simulink model "sampleModel7126_pp_difftest"  (R2018a)
settings: Solver=VariableStepAuto  StartTime=0.0  StopTime=10.0  RelTol=1e-3
undefined symbols (not defined in the file or in its folder): DiscIntNeverNeededParam
libraries: simulink x367
(part 1 of 8)
settings Model: Creator=cyfuzz  LastModifiedBy=verivitallab
settings CodeAppCC: StateflowObjectComments=on

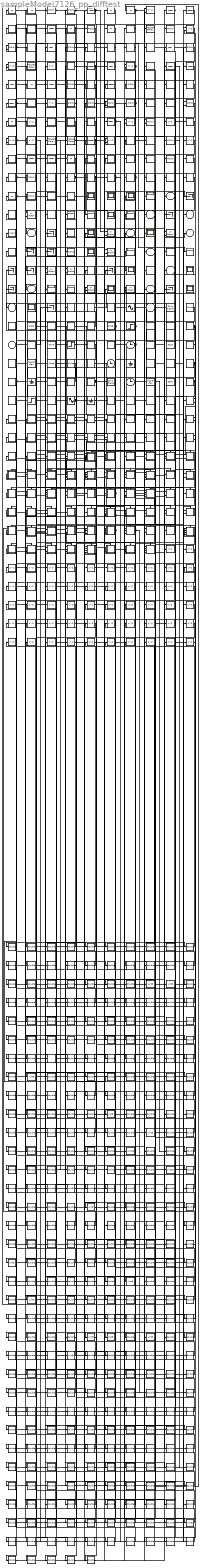
== system sampleModel7126_pp_difftest ==
  cfblk168 : Inport
  cfblk181 : Inport  Port=2
  cfblk{1..2,6..7,14,16,42,61,84,101} (10 alike) : UnitDelay
  cfblk{10,13,35,43,46,51,75,83} (8 alike) : DiscreteFilter  SampleTime=1
  cfblk{22,81,90,96..97,99..100,104} (8 alike) : simulink/Discrete/Difference  ICPrevInput=0.0  OutMin=[]  OutMax=[]  OutDataTypeStr=double  OutputDataTypeScalingMode=double  OutDataType=fixdt(1, 16)  OutScaling=2^-10  DoSatur=off
  cfblk{21,44,56,60,68,92,102} (7 alike) : simulink/Continuous/PID Controller (2DOF)  Controller=PID  TimeDomain=Discrete-time  SampleTime=1  IntegratorMethod=Forward Euler  FilterMethod=Forward Euler  Form=Parallel  UseFilter=on  ControllerParametersSource=internal  P=1  I=1  D=0  N=100  b=1  c=1  InitialConditionSource=internal  InitialConditionForIntegrator=0  InitialConditionForFilter=0  ExternalReset=none  LimitOutput=off  UpperSaturationLimit=inf  LowerSaturationLimit=-inf  LinearizeAsGain=off  AntiWindupMode=none  Kb=1  TrackingMode=off  Kt=1  PParamMin=[]  PParamMax=[]  IParamMin=[]  IParamMax=[]  DParamMin=[]  DParamMax=[]  NParamMin=[]  NParamMax=[]  bParamMin=[]  bParamMax=[]  cParamMin=[]  cParamMax=[]  KbParamMin=[]  KbParamMax=[]  KtParamMin=[]  KtParamMax=[]  POutMin=[]  POutMax=[]  IOutMin=[]  IOutMax=[]  DOutMin=[]  DOutMax=[]  NOutMin=[]  NOutMax=[]  bOutMin=[]  bOutMax=[]  cOutMin=[]  cOutMax=[]  KbOutMin=[]  KbOutMax=[]  KtOutMin=[]  KtOutMax=[]  IntegratorOutMin=[]  IntegratorOutMax=[]  FilterOutMin=[]  FilterOutMax=[]  SumOutMin=[]  SumOutMax=[]  Sum1OutMin=[]  Sum1OutMax=[]  Sum2OutMin=[]  Sum2OutMax=[]  Sum3OutMin=[]  Sum3OutMax=[]  SumI1OutMin=[]  SumI1OutMax=[]  SumI2OutMin=[]  SumI2OutMax=[]  SumI3OutMin=[]  SumI3OutMax=[]  SumDOutMin=[]  SumDOutMax=[]  SaturationOutMin=[]  SaturationOutMax=[]  IntegratorContinuousStateAttributes=''  IntegratorStateMustResolveToSignalObject=off  IntegratorRTWStateStorageClass=Auto  FilterContinuousStateAttributes=''  FilterStateMustResolveToSignalObject=off  FilterRTWStateStorageClass=Auto  DifferentiatorICPrevScaledInput=0  DifferentiatorOutMin=[]  DifferentiatorOutMax=[]  FilterDiffOutCoefMin=[]  FilterDiffOutCoefMax=[]  SumDenOutMin=[]  SumDenOutMax=[]  SumNumOutMin=[]  SumNumOutMax=[]  ReciprocalOutMin=[]  ReciprocalOutMax=[]  DivideOutMin=[]  DivideOutMax=[]  TunerSelectOption=Transfer Function Based (PID Tuner App)
  cfblk{25,52,58..59,64,103} (6 alike) : simulink/Discrete/Transfer Fcn Real Zero  ZeroZ=0.75  ICPrevInput=0.0  DoSatur=off
      settings: SourceProductName=Simulink  SourceProductBaseCode=SL
  cfblk{105..107,116,125,128,135,147,150,156,160,162} (12 alike) : Scope
      cfblk105 settings: Floating=on
      cfblk106 settings: Floating=on
      cfblk116 settings: Floating=on
      cfblk135 settings: Floating=on
      cfblk150 settings: Floating=on
      cfblk160 settings: Floating=on
      cfblk162 settings: Floating=on
  cfblk{108,114..115,117,137,140,153..154} (8 alike) : Display
  cfblk{11,27,45,49,85,93,95} (7 alike) : DiscreteStateSpace
  cfblk{110,119,123,132..133,141..142,146,151,159,163} (11 alike) : Terminator
  cfblk111 : ToWorkspace  VariableName=hcmzdjv  SaveFormat=Timeseries  SampleTime=-1
  cfblk{112,126,129,136,143..144,155,157} (8 alike) : simulink/Sinks/XY Graph  xmin=-1  xmax=1  ymin=-1  ymax=1  st=-1
  cfblk113 : ToWorkspace  VariableName=btwpcto  SaveFormat=Timeseries  SampleTime=-1
  cfblk{12,28,48,50,63,65,86,98} (8 alike) : DiscreteFir  SampleTime=1
  cfblk121 : ToWorkspace  VariableName=fvxrevr  SaveFormat=Timeseries  SampleTime=-1
  cfblk124 : ToWorkspace  VariableName=pxfsena  SaveFormat=Timeseries  SampleTime=-1
  cfblk131 : ToWorkspace  VariableName=uhzxskx  SaveFormat=Timeseries  SampleTime=-1
  cfblk134 : ToWorkspace  VariableName=rrjtpng  SaveFormat=Timeseries  SampleTime=-1
  cfblk139 : ToWorkspace  VariableName=kmkecre  SaveFormat=Timeseries  SampleTime=-1
  cfblk145 : ToWorkspace  VariableName=hvmekia  SaveFormat=Timeseries  SampleTime=-1
  cfblk148 : ToWorkspace  VariableName=eadgrso  SaveFormat=Timeseries  SampleTime=-1
  cfblk{3..4,15,19,24,30,47,54..55,57,79,89} (12 alike) : simulink/Continuous/PID Controller  Controller=PID  TimeDomain=Discrete-time  SampleTime=1  IntegratorMethod=Forward Euler  FilterMethod=Forward Euler  Form=Parallel  UseFilter=on  ControllerParametersSource=internal  P=1  I=1  D=0  N=100  InitialConditionSource=internal  InitialConditionForIntegrator=0  InitialConditionForFilter=0  ExternalReset=none  LimitOutput=off  UpperSaturationLimit=inf  LowerSaturationLimit=-inf  LinearizeAsGain=off  AntiWindupMode=none  Kb=1  TrackingMode=off  Kt=1  PParamMin=[]  PParamMax=[]  IParamMin=[]  IParamMax=[]  DParamMin=[]  DParamMax=[]  NParamMin=[]  NParamMax=[]  KbParamMin=[]  KbParamMax=[]  KtParamMin=[]  KtParamMax=[]  POutMin=[]  POutMax=[]  IOutMin=[]  IOutMax=[]  DOutMin=[]  DOutMax=[]  NOutMin=[]  NOutMax=[]  KbOutMin=[]  KbOutMax=[]  KtOutMin=[]  KtOutMax=[]  IntegratorOutMin=[]  IntegratorOutMax=[]  FilterOutMin=[]  FilterOutMax=[]  SumOutMin=[]  SumOutMax=[]  SumI1OutMin=[]  SumI1OutMax=[]  SumI2OutMin=[]  SumI2OutMax=[]  SumI3OutMin=[]  SumI3OutMax=[]  SumDOutMin=[]  SumDOutMax=[]  SaturationOutMin=[]  SaturationOutMax=[]  IntegratorContinuousStateAttributes=''  IntegratorStateMustResolveToSignalObject=off  IntegratorRTWStateStorageClass=Auto  FilterContinuousStateAttributes=''  FilterStateMustResolveToSignalObject=off  FilterRTWStateStorageClass=Auto  DifferentiatorICPrevScaledInput=0  DifferentiatorOutMin=[]  DifferentiatorOutMax=[]  FilterDiffOutCoefMin=[]  FilterDiffOutCoefMax=[]  SumDenOutMin=[]  SumDenOutMax=[]  SumNumOutMin=[]  SumNumOutMax=[]  ReciprocalOutMin=[]  ReciprocalOutMax=[]  DivideOutMin=[]  DivideOutMax=[]  TunerSelectOption=Transfer Function Based (PID Tuner App)
  cfblk164 : ToWorkspace  VariableName=thvkhab  SaveFormat=Timeseries  SampleTime=-1
  cfblk165 : simulink/Sources/Repeating Sequence Stair  OutValues=[3 1 4 2 1].'  tsamp=1  OutMin=[]  OutMax=[]  OutDataTypeStr=double  OutputDataTypeScalingMode=double  OutDataType=fixdt(0,8)  ConRadixGroup=Best Precision: Vector-wise  OutScaling=2^-12
  cfblk{166,174,180,213,216} (5 alike) : simulink/Sources/Repeating Sequence Interpolated  OutValues=[3 1 4 2 1].'  TimeValues=[0 0.1 0.5 0.6 1].'  LookUpMeth=Interpolation-Use End Values  tsamp=0.01  OutMin=[]  OutMax=[]  OutDataTypeStr=double  OutputDataTypeScalingMode=double  OutDataType=fixdt(0,8)  OutScaling=2^-10
  cfblk167 : Sin  SampleTime=0
  cfblk169 : simulink/Sources/Chirp Signal  f1=0.1  T=100  f2=1
  cfblk{17,38,87..88,91} (5 alike) : DiscreteZeroPole  Poles=[0 0.5]  Gain=1
  cfblk170 : DiscretePulseGenerator  PulseType=Time based  Period=10  PulseWidth=5
  cfblk{171,186,195,200,217} (5 alike) : simulink/Sources/Band-Limited White Noise  Cov=[0.1]  Ts=0.1  seed=[23341]
  cfblk172 : DigitalClock
  cfblk173 : RandomNumber  SampleTime=0.1
  cfblk{175,198..199,205,211} (5 alike) : simulink/Sources/Counter Free-Running  NumBits=16  tsamp=1
  cfblk176 : Constant  Value=0318  OutDataTypeStr=double  SampleTime=1
  cfblk177 : Step  After=82  SampleTime=0
  cfblk178 : simulink/Sources/Counter Limited  uplimit=7  tsamp=1
  cfblk179 : UniformRandomNumber  SampleTime=0.1
  cfblk{18,32,73..74} (4 alike) : simulink/Discrete/Tapped Delay  vinit=0.0  samptime=-1  NumDelays=1  DelayOrder=Oldest  includeCurrent=off
  cfblk182 : simulink/Sources/Repeating Sequence Stair  OutValues=[3 1 4 2 1].'  tsamp=1  OutMin=[]  OutMax=[]  OutDataTypeStr=double  OutputDataTypeScalingMode=double  OutDataType=fixdt(0,8)  ConRadixGroup=Best Precision: Vector-wise  OutScaling=2^-12
  cfblk183 : Constant  Value=5175  OutDataTypeStr=double  SampleTime=1
  cfblk184 : Step  After=84  SampleTime=0
  cfblk185 : simulink/Sources/Repeating Sequence  rep_seq_t=[0 2]  rep_seq_y=[0 2]
  cfblk187 : Clock
  cfblk188 : RandomNumber  SampleTime=0.1
  cfblk189 : Constant  Value=8152  OutDataTypeStr=double  SampleTime=1
  cfblk190 : simulink/Sources/Counter Limited  uplimit=7  tsamp=1
  cfblk191 : RandomNumber  SampleTime=0.1
  cfblk192 : SignalGenerator  Units=rad/sec
  cfblk193 : DiscretePulseGenerator  PulseType=Time based  Period=10  PulseWidth=5
  cfblk194 : DiscretePulseGenerator  PulseType=Time based  Period=10  PulseWidth=5
  cfblk196 : Clock
  cfblk197 : Ground
  cfblk20 : Delay  DelayLengthSource=Input port  SampleTime=1
      settings: InputPortMap=u0,p1
  cfblk201 : simulink/Sources/Repeating Sequence  rep_seq_t=[0 2]  rep_seq_y=[0 2]
  cfblk202 : Ground
  cfblk203 : simulink/Sources/Counter Limited  uplimit=7  tsamp=1
  cfblk204 : UniformRandomNumber  SampleTime=0.1
  cfblk206 : simulink/Sources/Chirp Signal  f1=0.1  T=100  f2=1
  cfblk207 : Clock
  cfblk208 : SignalGenerator  Units=rad/sec
  cfblk209 : Constant  Value=6334  OutDataTypeStr=double  SampleTime=1
  cfblk210 : UniformRandomNumber  SampleTime=0.1
  cfblk212 : Step  After=96  SampleTime=0
  cfblk214 : Sin  SampleTime=0
  cfblk215 : Ground
  cfblk{218..244} (27 alike) : If  SampleTime=1
  cfblk{23,29,36,41} (4 alike) : DiscreteIntegrator  OutDataTypeStr=double  ICPrevOutput=DiscIntNeverNeededParam  ICPrevScaledInput=DiscIntNeverNeededParam
  cfblk245 : Subsystem  TreatAsAtomicUnit=on
  cfblk246 : Subsystem  TreatAsAtomicUnit=on
  cfblk247 : Subsystem  TreatAsAtomicUnit=on
  cfblk248 : Subsystem  TreatAsAtomicUnit=on
  cfblk249 : Subsystem  TreatAsAtomicUnit=on
  cfblk250 : Subsystem  TreatAsAtomicUnit=on
  cfblk251 : Subsystem  TreatAsAtomicUnit=on
  cfblk252 : Subsystem  TreatAsAtomicUnit=on
  cfblk253 : Subsystem  TreatAsAtomicUnit=on
  cfblk254 : Subsystem  TreatAsAtomicUnit=on
  cfblk255 : Subsystem  TreatAsAtomicUnit=on
  cfblk256 : Subsystem  TreatAsAtomicUnit=on
  cfblk257 : Subsystem  TreatAsAtomicUnit=on
  cfblk258 : Subsystem  TreatAsAtomicUnit=on
  cfblk259 : Subsystem  TreatAsAtomicUnit=on
  cfblk{26,34,70,77} (4 alike) : simulink/Discrete/Transfer Fcn First Order  PoleZ=0.95  ICPrevOutput=0.0  DoSatur=off
      settings: SourceProductName=Simulink
  cfblk260 : Subsystem  TreatAsAtomicUnit=on
  cfblk261 : Subsystem  TreatAsAtomicUnit=on
  cfblk262 : Subsystem  TreatAsAtomicUnit=on
  cfblk263 : Subsystem  TreatAsAtomicUnit=on
  cfblk264 : Subsystem  TreatAsAtomicUnit=on
  cfblk265 : Subsystem  TreatAsAtomicUnit=on
  cfblk266 : Subsystem  TreatAsAtomicUnit=on
  cfblk267 : Subsystem  TreatAsAtomicUnit=on
  cfblk268 : Subsystem  TreatAsAtomicUnit=on
  cfblk269 : Subsystem  TreatAsAtomicUnit=on
  cfblk270 : Subsystem  TreatAsAtomicUnit=on
  cfblk271 : Subsystem  TreatAsAtomicUnit=on
  cfblk272 : Subsystem  TreatAsAtomicUnit=on
  cfblk273 : Subsystem  TreatAsAtomicUnit=on
  cfblk274 : Subsystem  TreatAsAtomicUnit=on
  cfblk275 : Subsystem  TreatAsAtomicUnit=on
  cfblk276 : Subsystem  TreatAsAtomicUnit=on
  cfblk277 : Subsystem  TreatAsAtomicUnit=on
  cfblk278 : Subsystem  TreatAsAtomicUnit=on
  cfblk279 : Subsystem  TreatAsAtomicUnit=on
  cfblk280 : Subsystem  TreatAsAtomicUnit=on
  cfblk281 : Subsystem  TreatAsAtomicUnit=on
  cfblk282 : Subsystem  TreatAsAtomicUnit=on
  cfblk283 : Subsystem  TreatAsAtomicUnit=on
  cfblk284 : Subsystem  TreatAsAtomicUnit=on
  cfblk285 : Subsystem  TreatAsAtomicUnit=on
  cfblk286 : Subsystem  TreatAsAtomicUnit=on
  cfblk287 : Subsystem  TreatAsAtomicUnit=on
  cfblk288 : Subsystem  TreatAsAtomicUnit=on
  cfblk289 : Subsystem  TreatAsAtomicUnit=on
  cfblk290 : Subsystem  TreatAsAtomicUnit=on
  cfblk291 : Subsystem  TreatAsAtomicUnit=on
  cfblk292 : Subsystem  TreatAsAtomicUnit=on
  cfblk293 : Subsystem  TreatAsAtomicUnit=on
  cfblk294 : Subsystem  TreatAsAtomicUnit=on
  cfblk295 : Subsystem  TreatAsAtomicUnit=on
  cfblk296 : Subsystem  TreatAsAtomicUnit=on
  cfblk297 : Subsystem  TreatAsAtomicUnit=on
  cfblk298 : Subsystem  TreatAsAtomicUnit=on
  cfblk{33,53,62,69,80,299..350} (57 alike) : Delay  SampleTime=1
  cfblk{31,37,67,72,76} (5 alike) : Delay  ShowEnablePort=on  SampleTime=1
      settings: InputPortMap=u0,e6
  cfblk{5,9,39..40,66,82} (6 alike) : DiscreteTransferFcn  SampleTime=1
  cfblk71 : Delay  DelayLengthSource=Input port  SampleTime=1
      settings: InputPortMap=u0,p1
  cfblk78 : simulink/Discrete/Transfer Fcn Lead or Lag  PoleZ=0.95  ZeroZ=0.75  ICPrevOutput=0.0  ICPrevInput=0.0  DoSatur=off
      settings: SourceProductName=Simulink  SourceProductBaseCode=SL
  cfblk8 : Delay  DelayLengthSource=Input port  SampleTime=1
      settings: InputPortMap=u0,p1
  cfblk94 : simulink/Discrete/Transfer Fcn Lead or Lag  PoleZ=0.95  ZeroZ=0.75  ICPrevOutput=0.0  ICPrevInput=0.0  DoSatur=off
      settings: SourceProductName=Simulink  SourceProductBaseCode=SL
  cyemi_{0..26,29..61,63..67,99..100,133,181,203..205,222..224,233,243,297..298,328..331,345..348,357..358,383..384,395..398,407,446..448,457,485..486,496..498,533..534,548,589,615,629..632,639..640,673..674,688..689,706,719..720,753,763,802..803,813..814,856..857,929..930,939,941,971..973,985..987,999..1000,1013..1014,1055..1057,1064..1065,1070..1072,1081..1082,1094,1133,1136..1137,1146,1154..1155,1186..1187,1202..1204,1216..1219,1266,1285..1287,1295,1297..1298,1340..1359,1362,1364..1367,1370..1409,1411..1430,1432..1464,1466..1480} (311 alike) : DataTypeConversion  OutDataTypeStr=double
  cyemi_{27..28,180,385,495,801,940,1063,1135,1267,1296,1360..1361,1363,1369,1410,1465} (17 alike) : DataTypeConversion  OutDataTypeStr=uint8
  cyemi_{616,707,804,1134,1431} (5 alike) : DataTypeConversion  OutDataTypeStr=uint16
  cyemi_1368 : DataTypeConversion  OutDataTypeStr=fixdt('ufix32_En8')
  cyemi_62 : DataTypeConversion  OutDataTypeStr=fixdt('ufix32_En8')
  cfblk109 : Outport
  cfblk118 : Outport  Port=2
  cfblk120 : Outport  Port=3
  cfblk122 : Outport  Port=4
  cfblk127 : Outport  Port=5
  cfblk130 : Outport  Port=6
  cfblk138 : Outport  Port=7
  cfblk149 : Outport  Port=8
  cfblk152 : Outport  Port=9
  cfblk158 : Outport  Port=10
  cfblk161 : Outport  Port=11
  wires:
  cfblk249/1(cfblk2) -> cfblk149/1
  cfblk21/1 -> cfblk147/1, cyemi_53/1
  cfblk182/1 -> cfblk163/1
  cfblk11/1 -> cfblk140/1
  cfblk269/2(cfblk7) -> cyemi_689/1, cyemi_1370/1, cyemi_1459/1
  cfblk34/1 -> cfblk118/1
  cfblk175/1 -> cfblk153/1
  cfblk13/1 -> cfblk119/1
  cfblk211/1 -> cfblk108/1
  cfblk4/1 -> cyemi_719/1, cyemi_814/1, cyemi_1441/1
  cfblk252/1(cfblk2) -> cyemi_1383/1, cyemi_1468/1
  cfblk286/1(cfblk2) -> cyemi_1360/1, cyemi_1369/1
  cfblk180/1 -> cyemi_1365/1, cyemi_1476/1
  cfblk23/1 -> cyemi_1136/1, cyemi_1397/1, cyemi_1406/1
  cfblk268/1(cfblk2) -> cfblk109/1
  cfblk282/1(cfblk2) -> cfblk123/1
  cfblk14/1 -> cyemi_99/1, cyemi_986/1
  cfblk75/1 -> cfblk110/1, cyemi_1409/1
  cfblk9/1 -> cyemi_534/1, cyemi_1392/1
  cfblk101/1 -> cfblk136/2, cyemi_1351/1
  cfblk51/1 -> cyemi_397/1, cyemi_1384/1, cyemi_1471/1
  cfblk95/1 -> cyemi_1376/1, cyemi_1442/1
  cfblk178/1 -> cyemi_385/1, cyemi_940/1
  cfblk37/1 -> cfblk112/1, cfblk126/2, cyemi_1347/1
  cfblk177/1 -> cyemi_1432/1, cyemi_1452/1
  cfblk254/1(cfblk2) -> cfblk144/1
  cfblk200/1 -> cyemi_17/1, cyemi_803/1
  cfblk268/3(cfblk13) -> cfblk130/1, cyemi_1402/1
  cfblk59/1 -> cyemi_25/1, cyemi_133/1
  cfblk87/1 -> cfblk115/1
  cfblk53/1 -> cyemi_14/1, cyemi_1344/1
  cfblk71/1 -> cyemi_37/1, cyemi_448/1, cyemi_1340/1
  cfblk188/1 -> cfblk159/1
  cfblk62/1 -> cfblk142/1
  cfblk73/1 -> cfblk129/2, cyemi_673/1
  cfblk66/1 -> cyemi_6/1, cyemi_31/1, cyemi_1440/1
  cfblk166/1 -> cfblk138/1
  cfblk3/1 -> cyemi_65/1, cyemi_1443/1
  cfblk7/1 -> cyemi_18/1, cyemi_56/1
  cfblk287/1(cfblk2) -> cyemi_3/1, cyemi_987/1, cyemi_1393/1
  cfblk266/1(cfblk2) -> cyemi_1378/1, cyemi_1379/1
  cfblk48/1 -> cyemi_589/1, cyemi_1380/1
  cfblk72/1 -> cyemi_1346/1, cyemi_1348/1
  cfblk278/1(cfblk2) -> cfblk107/1
  cfblk214/1 -> cfblk114/1, cyemi_331/1
  cfblk176/1 -> cyemi_1000/1, cyemi_1401/1
  cfblk263/2(cfblk14) -> cfblk143/1
  cfblk172/1 -> cyemi_486/1, cyemi_1297/1
  cfblk91/1 -> cfblk161/1, cyemi_222/1
  cfblk283/1(cfblk2) -> cfblk143/2
  cfblk100/1 -> cfblk112/2
  cfblk261/1(cfblk2) -> cfblk137/1
  cfblk277/2(cfblk17) -> cfblk125/1
  cfblk210/1 -> cyemi_1070/1, cyemi_1436/1
  cfblk187/1 -> cfblk141/1, cyemi_1341/1
  cfblk281/1(cfblk2) -> cfblk127/1
  cfblk205/1 -> cyemi_616/1, cyemi_804/1
  cfblk206/1 -> cfblk154/1
  cfblk57/1 -> cfblk122/1, cyemi_45/1
  cfblk5/1 -> cfblk126/1, cyemi_857/1
  cfblk64/1 -> cfblk132/1
  cfblk204/1 -> cfblk133/1
  cfblk253/1(cfblk2) -> cfblk158/1
  cfblk94/1 -> cyemi_15/1, cyemi_383/1
  cfblk39/1 -> cyemi_328/1, cyemi_497/1
  cfblk247/3(cfblk17) -> cfblk117/1
  cfblk35/1 -> cyemi_59/1, cyemi_498/1
  cfblk183/1 -> cyemi_396/1, cyemi_1056/1
  cfblk201/1 -> cyemi_447/1, cyemi_1014/1
  cfblk250/2(cfblk9) -> cyemi_1071/1, cyemi_1155/1
  cfblk280/3(cfblk12) -> cfblk155/1
  cfblk208/1 -> cyemi_630/1, cyemi_1420/1
  cfblk168/1 -> cyemi_348/1, cyemi_398/1
  cfblk248/2(cfblk17) -> cyemi_446/1, cyemi_1154/1
  cfblk83/1 -> cyemi_813/1, cyemi_1371/1
  cfblk25/1 -> cfblk136/1
  cfblk251/1(cfblk2) -> cfblk155/2
  cfblk79/1 -> cyemi_496/1, cyemi_1435/1
  cfblk276/3(cfblk13) -> cyemi_1134/1, cyemi_1431/1
  cfblk96/1 -> cyemi_330/1, cyemi_1472/1
  cfblk207/1 -> cfblk129/1
  cfblk15/1 -> cfblk152/1
  cfblk199/1 -> cfblk120/1
  cfblk165/1 -> cfblk157/1
  cfblk296/3(cfblk17) -> cfblk146/1
  cfblk97/1 -> cyemi_457/1, cyemi_1446/1
  cfblk289/2(cfblk8) -> cfblk157/2, cyemi_1394/1
  cfblk292/3(cfblk13) -> cfblk151/1, cyemi_243/1
  cfblk290/4(cfblk15) -> cfblk156/1
  cfblk283/4(cfblk17) -> cyemi_181/1, cyemi_1385/1
  cfblk264/3(cfblk14) -> cfblk128/1
  cfblk288/1(cfblk2) -> cyemi_1366/1, cyemi_1367/1
  cfblk297/2(cfblk10) -> cfblk144/2
  cfblk218/1 -> cfblk245/Action
  cfblk218/2 -> cfblk246/Action
  cfblk219/1 -> cfblk247/Action
  cfblk219/2 -> cfblk248/Action
  cfblk220/1 -> cfblk249/Action
  cfblk220/2 -> cfblk250/Action
  cfblk221/1 -> cfblk251/Action
  cfblk221/2 -> cfblk252/Action
  cfblk222/1 -> cfblk253/Action
  cfblk222/2 -> cfblk254/Action
  cfblk223/1 -> cfblk255/Action
  cfblk223/2 -> cfblk256/Action
  cfblk224/1 -> cfblk257/Action
  cfblk224/2 -> cfblk258/Action
  cfblk225/1 -> cfblk259/Action
  cfblk225/2 -> cfblk260/Action
  cfblk226/1 -> cfblk261/Action
  cfblk226/2 -> cfblk262/Action
  cfblk227/1 -> cfblk263/Action
  cfblk227/2 -> cfblk264/Action
  cfblk228/1 -> cfblk265/Action
  cfblk228/2 -> cfblk266/Action
  cfblk229/1 -> cfblk267/Action
  cfblk229/2 -> cfblk268/Action
  cfblk230/1 -> cfblk269/Action
  cfblk230/2 -> cfblk270/Action
  cfblk231/1 -> cfblk271/Action
  cfblk231/2 -> cfblk272/Action
  cfblk232/1 -> cfblk273/Action
  cfblk232/2 -> cfblk274/Action
  cfblk233/1 -> cfblk275/Action
  cfblk233/2 -> cfblk276/Action
  cfblk234/1 -> cfblk277/Action
  cfblk234/2 -> cfblk278/Action
  cfblk235/1 -> cfblk279/Action
  cfblk235/2 -> cfblk280/Action
  cfblk236/1 -> cfblk281/Action
  cfblk236/2 -> cfblk282/Action
  cfblk237/1 -> cfblk283/Action
  cfblk237/2 -> cfblk284/Action
  cfblk238/1 -> cfblk285/Action
  cfblk238/2 -> cfblk286/Action
  cfblk239/1 -> cfblk287/Action
  cfblk239/2 -> cfblk288/Action
  cfblk240/1 -> cfblk289/Action
  cfblk240/2 -> cfblk290/Action
  cfblk241/1 -> cfblk291/Action
  cfblk241/2 -> cfblk292/Action
  cfblk242/1 -> cfblk293/Action
  cfblk242/2 -> cfblk294/Action
  cfblk243/1 -> cfblk295/Action
  cfblk243/2 -> cfblk296/Action
  cfblk244/1 -> cfblk297/Action
  cfblk244/2 -> cfblk298/Action
  cyemi_0/1 -> cfblk1/1
  cfblk290/5(cfblk16) -> cyemi_0/1
  cyemi_1/1 -> cfblk10/1
  cfblk196/1 -> cyemi_1/1
  cyemi_2/1 -> cfblk100/1
  cfblk33/1 -> cyemi_2/1
  cyemi_3/1 -> cfblk101/1
  cyemi_4/1 -> cfblk102/1
  cfblk282/5(cfblk15) -> cyemi_4/1
  cyemi_5/1 -> cfblk102/2
  cfblk16/1 -> cyemi_5/1
  cyemi_6/1 -> cfblk103/1
  cyemi_7/1 -> cfblk104/1
  cfblk267/2(cfblk14) -> cyemi_7/1
  cyemi_8/1 -> cfblk11/1
  cfblk259/2(cfblk8) -> cyemi_8/1
  cyemi_9/1 -> cfblk111/1
  cfblk257/1(cfblk2) -> cyemi_9/1
  cyemi_10/1 -> cfblk113/1
  cfblk171/1 -> cyemi_10/1
  cyemi_11/1 -> cfblk12/1
  cfblk40/1 -> cyemi_11/1
  cyemi_12/1 -> cfblk121/1
  cfblk194/1 -> cyemi_12/1
  cyemi_13/1 -> cfblk124/1
  cfblk80/1 -> cyemi_13/1
  cyemi_14/1 -> cfblk13/1
  cyemi_15/1 -> cfblk131/1
  cyemi_16/1 -> cfblk134/1
  cfblk268/2(cfblk12) -> cyemi_16/1
  cyemi_17/1 -> cfblk139/1
  cyemi_18/1 -> cfblk14/1
  cyemi_19/1 -> cfblk145/1
  cfblk248/1(cfblk2) -> cyemi_19/1
  cyemi_20/1 -> cfblk148/1
  cfblk26/1 -> cyemi_20/1
  cyemi_21/1 -> cfblk15/1
  cfblk298/1(cfblk2) -> cyemi_21/1
  cyemi_22/1 -> cfblk16/1
  cfblk47/1 -> cyemi_22/1
  cyemi_23/1 -> cfblk164/1
  cfblk247/1(cfblk2) -> cyemi_23/1
  cyemi_24/1 -> cfblk17/1
  cfblk272/1(cfblk2) -> cyemi_24/1
  cyemi_25/1 -> cfblk18/1
  cyemi_26/1 -> cfblk19/1
  cfblk202/1 -> cyemi_26/1
  cyemi_27/1 -> cfblk2/1
  cfblk318/1 -> cyemi_27/1
  cyemi_28/1 -> cfblk20/1
  cfblk2/1 -> cyemi_28/1
  cyemi_29/1 -> cfblk20/2
  cfblk350/1 -> cyemi_29/1
  cyemi_30/1 -> cfblk21/1
  cfblk259/1(cfblk2) -> cyemi_30/1
  cyemi_31/1 -> cfblk21/2
  cyemi_32/1 -> cfblk218/1
  cfblk300/1 -> cyemi_32/1
  cyemi_33/1 -> cfblk219/1
  cfblk63/1 -> cyemi_33/1
  cyemi_34/1 -> cfblk22/1
  cfblk181/1 -> cyemi_34/1
  cyemi_35/1 -> cfblk220/1
  cfblk293/1(cfblk2) -> cyemi_35/1
  cyemi_36/1 -> cfblk221/1
  cfblk61/1 -> cyemi_36/1
  cyemi_37/1 -> cfblk222/1
  cyemi_38/1 -> cfblk223/1
  cfblk306/1 -> cyemi_38/1
  cyemi_39/1 -> cfblk224/1
  cfblk28/1 -> cyemi_39/1
  cyemi_40/1 -> cfblk225/1
  cfblk317/1 -> cyemi_40/1
  cyemi_41/1 -> cfblk226/1
  cfblk88/1 -> cyemi_41/1
  cyemi_42/1 -> cfblk227/1
  cfblk70/1 -> cyemi_42/1
  cyemi_43/1 -> cfblk228/1
  cfblk27/1 -> cyemi_43/1
  cyemi_44/1 -> cfblk229/1
  cfblk303/1 -> cyemi_44/1
  cyemi_45/1 -> cfblk23/1
  cyemi_46/1 -> cfblk230/1
  cfblk325/1 -> cyemi_46/1
  cyemi_47/1 -> cfblk231/1
  cfblk284/2(cfblk9) -> cyemi_47/1
  cyemi_48/1 -> cfblk232/1
  cfblk311/1 -> cyemi_48/1
  cyemi_49/1 -> cfblk233/1
  cfblk191/1 -> cyemi_49/1
  cyemi_50/1 -> cfblk234/1
  cfblk84/1 -> cyemi_50/1
  cyemi_51/1 -> cfblk235/1
  cfblk93/1 -> cyemi_51/1
  cyemi_52/1 -> cfblk236/1
  cfblk60/1 -> cyemi_52/1
  cyemi_53/1 -> cfblk237/1
  cyemi_54/1 -> cfblk238/1
  cfblk314/1 -> cyemi_54/1
  cyemi_55/1 -> cfblk239/1
  cfblk340/1 -> cyemi_55/1
  cyemi_56/1 -> cfblk24/1
  cyemi_57/1 -> cfblk240/1
  cfblk313/1 -> cyemi_57/1
  cyemi_58/1 -> cfblk241/1
  cfblk329/1 -> cyemi_58/1
  cyemi_59/1 -> cfblk242/1
  cyemi_60/1 -> cfblk243/1
  cfblk245/3(cfblk17) -> cyemi_60/1
  cyemi_61/1 -> cfblk244/1
  cfblk285/1(cfblk2) -> cyemi_61/1
  cyemi_62/1 -> cfblk245/1(cfblk1)
  cfblk322/1 -> cyemi_62/1
  cyemi_63/1 -> cfblk245/2(cfblk11)
  cfblk320/1 -> cyemi_63/1
  cyemi_64/1 -> cfblk245/3(cfblk12)
  cfblk260/2(cfblk10) -> cyemi_64/1
  cyemi_65/1 -> cfblk245/4(cfblk13)
  cyemi_66/1 -> cfblk245/5(cfblk14)
  cfblk333/1 -> cyemi_66/1
  cyemi_67/1 -> cfblk245/6(cfblk15)
  cfblk345/1 -> cyemi_67/1
  cyemi_99/1 -> cfblk246/1(cfblk1)
  cyemi_100/1 -> cfblk246/2(cfblk8)
  cfblk52/1 -> cyemi_100/1
  cyemi_133/1 -> cfblk247/1(cfblk1)
  cyemi_180/1 -> cfblk248/1(cfblk1)
  cfblk276/2(cfblk12) -> cyemi_180/1
  cyemi_181/1 -> cfblk248/2(cfblk16)
  cyemi_203/1 -> cfblk249/1(cfblk1)
  cfblk54/1 -> cyemi_203/1
  cyemi_204/1 -> cfblk249/2(cfblk14)
  cfblk10/1 -> cyemi_204/1
  cyemi_205/1 -> cfblk249/3(cfblk15)
  cfblk341/1 -> cyemi_205/1
  cyemi_222/1 -> cfblk25/1
  cyemi_223/1 -> cfblk250/1(cfblk1)
  cfblk184/1 -> cyemi_223/1
  cyemi_224/1 -> cfblk250/2(cfblk8)
  cfblk305/1 -> cyemi_224/1
  cyemi_233/1 -> cfblk251/1(cfblk1)
  cfblk292/2(cfblk12) -> cyemi_233/1
  cyemi_243/1 -> cfblk252/1(cfblk1)
  cyemi_297/1 -> cfblk253/1(cfblk1)
  cfblk261/2(cfblk12) -> cyemi_297/1
  cyemi_298/1 -> cfblk253/2(cfblk8)
  cfblk274/2(cfblk8) -> cyemi_298/1
  cyemi_328/1 -> cfblk254/1(cfblk1)
  cyemi_329/1 -> cfblk254/2(cfblk14)
  cfblk255/1(cfblk2) -> cyemi_329/1
  cyemi_330/1 -> cfblk254/3(cfblk15)
  cyemi_331/1 -> cfblk254/4(cfblk16)
  cyemi_345/1 -> cfblk255/1(cfblk1)
  cfblk343/1 -> cyemi_345/1
  cyemi_346/1 -> cfblk255/2(cfblk9)
  cfblk339/1 -> cyemi_346/1
  cyemi_347/1 -> cfblk255/3(cfblk10)
  cfblk267/1(cfblk2) -> cyemi_347/1
  cyemi_348/1 -> cfblk255/4(cfblk11)
  cyemi_357/1 -> cfblk256/1(cfblk1)
  cfblk330/1 -> cyemi_357/1
  cyemi_358/1 -> cfblk256/2(cfblk10)
  cfblk307/1 -> cyemi_358/1
  cyemi_383/1 -> cfblk257/1(cfblk1)
  cyemi_384/1 -> cfblk257/2(cfblk12)
  cfblk264/2(cfblk13) -> cyemi_384/1
  cyemi_385/1 -> cfblk257/3(cfblk13)
  cyemi_395/1 -> cfblk258/1(cfblk1)
  cfblk56/1 -> cyemi_395/1
  cyemi_396/1 -> cfblk258/2(cfblk8)
  cyemi_397/1 -> cfblk258/3(cfblk9)
  cyemi_398/1 -> cfblk258/4(cfblk10)
  cyemi_407/1 -> cfblk259/1(cfblk1)
  cfblk308/1 -> cyemi_407/1
  cyemi_446/1 -> cfblk26/1
  cyemi_447/1 -> cfblk260/1(cfblk1)
  cyemi_448/1 -> cfblk260/2(cfblk9)
  cyemi_457/1 -> cfblk261/1(cfblk1)
  cyemi_485/1 -> cfblk262/1(cfblk1)
  cfblk197/1 -> cyemi_485/1
  cyemi_486/1 -> cfblk262/2(cfblk9)
  cyemi_495/1 -> cfblk263/1(cfblk1)
  cfblk280/2(cfblk11) -> cyemi_495/1
  cyemi_496/1 -> cfblk263/2(cfblk11)
  cyemi_497/1 -> cfblk263/3(cfblk12)
  cyemi_498/1 -> cfblk263/4(cfblk13)
  cyemi_533/1 -> cfblk264/1(cfblk1)
  cfblk256/1(cfblk2) -> cyemi_533/1
  cyemi_534/1 -> cfblk264/2(cfblk12)
  cyemi_548/1 -> cfblk265/1(cfblk1)
  cfblk50/1 -> cyemi_548/1
  cyemi_589/1 -> cfblk266/1(cfblk1)
  cyemi_615/1 -> cfblk267/1(cfblk1)
  cfblk46/1 -> cyemi_615/1
  cyemi_616/1 -> cfblk267/2(cfblk13)
  cyemi_629/1 -> cfblk268/1(cfblk1)
  cfblk334/1 -> cyemi_629/1
  cyemi_630/1 -> cfblk268/2(cfblk9)
  cyemi_631/1 -> cfblk268/3(cfblk10)
  cfblk338/1 -> cyemi_631/1
  cyemi_632/1 -> cfblk268/4(cfblk11)
  cfblk304/1 -> cyemi_632/1
  cyemi_639/1 -> cfblk269/1(cfblk1)
  cfblk32/1 -> cyemi_639/1
  cyemi_640/1 -> cfblk269/2(cfblk6)
  cfblk331/1 -> cyemi_640/1
  cyemi_673/1 -> cfblk27/1
  cyemi_674/1 -> cfblk270/1(cfblk1)
  cfblk292/1(cfblk2) -> cyemi_674/1
  cyemi_688/1 -> cfblk271/1(cfblk1)
  cfblk174/1 -> cyemi_688/1
  cyemi_689/1 -> cfblk271/2(cfblk14)
  cyemi_706/1 -> cfblk272/1(cfblk1)
  cfblk344/1 -> cyemi_706/1
  cyemi_707/1 -> cfblk272/2(cfblk9)
  cfblk198/1 -> cyemi_707/1
  cyemi_719/1 -> cfblk273/1(cfblk1)
  cyemi_720/1 -> cfblk273/2(cfblk8)
  cfblk45/1 -> cyemi_720/1
  cyemi_753/1 -> cfblk274/1(cfblk1)
  cfblk264/1(cfblk2) -> cyemi_753/1
  cyemi_763/1 -> cfblk275/1(cfblk1)
  cfblk336/1 -> cyemi_763/1
  cyemi_801/1 -> cfblk276/1(cfblk1)
  cfblk20/1 -> cyemi_801/1
  cyemi_802/1 -> cfblk276/2(cfblk9)
  cfblk301/1 -> cyemi_802/1
  cyemi_803/1 -> cfblk276/3(cfblk10)
  cyemi_804/1 -> cfblk276/4(cfblk11)
  cyemi_813/1 -> cfblk277/1(cfblk1)
  cyemi_814/1 -> cfblk277/2(cfblk16)
  cyemi_856/1 -> cfblk278/1(cfblk1)
  cfblk69/1 -> cyemi_856/1
  cyemi_857/1 -> cfblk278/2(cfblk10)
  cyemi_929/1 -> cfblk279/1(cfblk1)
  cfblk271/1(cfblk2) -> cyemi_929/1
  cyemi_930/1 -> cfblk279/2(cfblk8)
  cfblk283/3(cfblk16) -> cyemi_930/1
  cyemi_939/1 -> cfblk28/1
  cfblk273/1(cfblk2) -> cyemi_939/1
  cyemi_940/1 -> cfblk280/1(cfblk1)
  cyemi_941/1 -> cfblk280/2(cfblk10)
  cfblk104/1 -> cyemi_941/1
  cyemi_971/1 -> cfblk281/1(cfblk1)
  cfblk55/1 -> cyemi_971/1
  cyemi_972/1 -> cfblk281/2(cfblk12)
  cfblk192/1 -> cyemi_972/1
  cyemi_973/1 -> cfblk281/3(cfblk13)
  cfblk251/2(cfblk11) -> cyemi_973/1
  cyemi_985/1 -> cfblk282/1(cfblk1)
  cfblk74/1 -> cyemi_985/1
  cyemi_986/1 -> cfblk282/2(cfblk10)
  cyemi_987/1 -> cfblk282/3(cfblk11)
  cyemi_999/1 -> cfblk283/1(cfblk1)
  cfblk324/1 -> cyemi_999/1
  cyemi_1000/1 -> cfblk283/2(cfblk14)
  cyemi_1013/1 -> cfblk284/1(cfblk1)
  cfblk170/1 -> cyemi_1013/1
  cyemi_1014/1 -> cfblk284/2(cfblk8)
  cyemi_1055/1 -> cfblk285/1(cfblk1)
  cfblk276/1(cfblk2) -> cyemi_1055/1
  cyemi_1056/1 -> cfblk285/2(cfblk8)
  cyemi_1057/1 -> cfblk285/3(cfblk9)
  cfblk346/1 -> cyemi_1057/1
  cyemi_1063/1 -> cfblk286/1(cfblk1)
  cfblk190/1 -> cyemi_1063/1
  cyemi_1064/1 -> cfblk286/2(cfblk7)
  cfblk179/1 -> cyemi_1064/1
  cyemi_1065/1 -> cfblk286/3(cfblk8)
  cfblk337/1 -> cyemi_1065/1
  cyemi_1070/1 -> cfblk287/1(cfblk1)
  cyemi_1071/1 -> cfblk287/2(cfblk8)
  cyemi_1072/1 -> cfblk287/3(cfblk9)
  cfblk328/1 -> cyemi_1072/1
  cyemi_1081/1 -> cfblk288/1(cfblk1)
  cfblk212/1 -> cyemi_1081/1
  cyemi_1082/1 -> cfblk288/2(cfblk13)
  cfblk319/1 -> cyemi_1082/1
  cyemi_1094/1 -> cfblk289/1(cfblk1)
  cfblk44/1 -> cyemi_1094/1
  cyemi_1133/1 -> cfblk29/1
  cfblk277/1(cfblk2) -> cyemi_1133/1
  cyemi_1134/1 -> cfblk290/1(cfblk1)
  cyemi_1135/1 -> cfblk290/2(cfblk10)
  cfblk323/1 -> cyemi_1135/1
  cyemi_1136/1 -> cfblk290/3(cfblk11)
  cyemi_1137/1 -> cfblk290/4(cfblk12)
  cfblk321/1 -> cyemi_1137/1
  cyemi_1146/1 -> cfblk291/1(cfblk1)
  cfblk332/1 -> cyemi_1146/1
  cyemi_1154/1 -> cfblk292/1(cfblk1)
  cyemi_1155/1 -> cfblk292/2(cfblk11)
  cyemi_1186/1 -> cfblk293/1(cfblk1)
  cfblk216/1 -> cyemi_1186/1
  cyemi_1187/1 -> cfblk293/2(cfblk9)
  cfblk169/1 -> cyemi_1187/1
  cyemi_1202/1 -> cfblk294/1(cfblk1)
  cfblk310/1 -> cyemi_1202/1
  cyemi_1203/1 -> cfblk294/2(cfblk9)
  cfblk217/1 -> cyemi_1203/1
  cyemi_1204/1 -> cfblk294/3(cfblk10)
  cfblk342/1 -> cyemi_1204/1
  cyemi_1216/1 -> cfblk295/1(cfblk1)
  cfblk326/1 -> cyemi_1216/1
  cyemi_1217/1 -> cfblk295/2(cfblk9)
  cfblk327/1 -> cyemi_1217/1
  cyemi_1218/1 -> cfblk295/3(cfblk10)
  cfblk309/1 -> cyemi_1218/1
  cyemi_1219/1 -> cfblk295/4(cfblk11)
  cfblk260/3(cfblk11) -> cyemi_1219/1
  cyemi_1266/1 -> cfblk296/1(cfblk1)
  cfblk103/1 -> cyemi_1266/1
  cyemi_1267/1 -> cfblk296/2(cfblk15)
  cfblk315/1 -> cyemi_1267/1
  cyemi_1285/1 -> cfblk297/1(cfblk1)
  cfblk302/1 -> cyemi_1285/1
  cyemi_1286/1 -> cfblk297/2(cfblk8)
  cfblk299/1 -> cyemi_1286/1
  cyemi_1287/1 -> cfblk297/3(cfblk9)
  cfblk349/1 -> cyemi_1287/1
  cyemi_1295/1 -> cfblk298/1(cfblk1)
  cfblk348/1 -> cyemi_1295/1
  cyemi_1296/1 -> cfblk298/2(cfblk9)
  cfblk316/1 -> cyemi_1296/1
  cyemi_1297/1 -> cfblk298/3(cfblk10)
  cyemi_1298/1 -> cfblk298/4(cfblk11)
  cfblk347/1 -> cyemi_1298/1
  cyemi_1340/1 -> cfblk299/1
  cyemi_1341/1 -> cfblk3/1
  cyemi_1342/1 -> cfblk30/1
  cfblk173/1 -> cyemi_1342/1
  cyemi_1343/1 -> cfblk300/1
  cfblk81/1 -> cyemi_1343/1
  cyemi_1344/1 -> cfblk301/1
  cyemi_1345/1 -> cfblk302/1
  cfblk245/2(cfblk16) -> cyemi_1345/1
  cyemi_1346/1 -> cfblk303/1
  cyemi_1347/1 -> cfblk304/1
  cyemi_1348/1 -> cfblk305/1
  cyemi_1349/1 -> cfblk306/1
  cfblk250/1(cfblk2) -> cyemi_1349/1
  cyemi_1350/1 -> cfblk307/1
  cfblk257/2(cfblk14) -> cyemi_1350/1
  cyemi_1351/1 -> cfblk308/1
  cyemi_1352/1 -> cfblk309/1
  cfblk283/2(cfblk15) -> cyemi_1352/1
  cyemi_1353/1 -> cfblk31/1
  cfblk247/2(cfblk16) -> cyemi_1353/1
  cyemi_1354/1 -> cfblk31/2
  cfblk260/4(cfblk12) -> cyemi_1354/1
  cyemi_1355/1 -> cfblk310/1
  cfblk258/1(cfblk2) -> cyemi_1355/1
  cyemi_1356/1 -> cfblk311/1
  cfblk294/1(cfblk2) -> cyemi_1356/1
  cyemi_1357/1 -> cfblk312/1
  cfblk6/1 -> cyemi_1357/1
  cyemi_1358/1 -> cfblk313/1
  cfblk270/1(cfblk2) -> cyemi_1358/1
  cyemi_1359/1 -> cfblk314/1
  cfblk269/1(cfblk2) -> cyemi_1359/1
  cyemi_1360/1 -> cfblk315/1
  cyemi_1361/1 -> cfblk316/1
  cfblk296/1(cfblk2) -> cyemi_1361/1
  cyemi_1362/1 -> cfblk317/1
  cfblk298/2(cfblk12) -> cyemi_1362/1
  cyemi_1363/1 -> cfblk318/1
  cfblk298/3(cfblk13) -> cyemi_1363/1
  cyemi_1364/1 -> cfblk319/1
  cfblk298/4(cfblk14) -> cyemi_1364/1
  cyemi_1365/1 -> cfblk32/1
  cyemi_1366/1 -> cfblk320/1
  cyemi_1367/1 -> cfblk321/1
  cyemi_1368/1 -> cfblk322/1
  cfblk86/1 -> cyemi_1368/1
  cyemi_1369/1 -> cfblk323/1
  cyemi_1370/1 -> cfblk324/1
  cyemi_1371/1 -> cfblk325/1
  cyemi_1372/1 -> cfblk326/1
  cfblk291/1(cfblk2) -> cyemi_1372/1
  cyemi_1373/1 -> cfblk327/1
  cfblk90/1 -> cyemi_1373/1
  cyemi_1374/1 -> cfblk328/1
  cfblk265/2(cfblk8) -> cyemi_1374/1
  cyemi_1375/1 -> cfblk329/1
  cfblk29/1 -> cyemi_1375/1
  cyemi_1376/1 -> cfblk33/1
  cyemi_1377/1 -> cfblk330/1
  cfblk38/1 -> cyemi_1377/1
  cyemi_1378/1 -> cfblk331/1
  cyemi_1379/1 -> cfblk332/1
  cyemi_1380/1 -> cfblk333/1
  cyemi_1381/1 -> cfblk334/1
  cfblk262/2(cfblk10) -> cyemi_1381/1
  cyemi_1382/1 -> cfblk335/1
  cfblk89/1 -> cyemi_1382/1
  cyemi_1383/1 -> cfblk336/1
  cyemi_1384/1 -> cfblk337/1
  cyemi_1385/1 -> cfblk338/1
  cyemi_1386/1 -> cfblk339/1
  cfblk282/2(cfblk12) -> cyemi_1386/1
  cyemi_1387/1 -> cfblk34/1
  cfblk99/1 -> cyemi_1387/1
  cyemi_1388/1 -> cfblk340/1
  cfblk282/3(cfblk13) -> cyemi_1388/1
  cyemi_1389/1 -> cfblk341/1
  cfblk282/4(cfblk14) -> cyemi_1389/1
  cyemi_1390/1 -> cfblk342/1
  cfblk102/1 -> cyemi_1390/1
  cyemi_1391/1 -> cfblk343/1
  cfblk98/1 -> cyemi_1391/1
  cyemi_1392/1 -> cfblk344/1
  cyemi_1393/1 -> cfblk345/1
  cyemi_1394/1 -> cfblk346/1
  cyemi_1395/1 -> cfblk347/1
  cfblk255/3(cfblk13) -> cyemi_1395/1
  cyemi_1396/1 -> cfblk348/1
  cfblk280/1(cfblk2) -> cyemi_1396/1
  cyemi_1397/1 -> cfblk349/1
  cyemi_1398/1 -> cfblk35/1
  cfblk255/2(cfblk12) -> cyemi_1398/1
  cyemi_1399/1 -> cfblk350/1
  cfblk295/2(cfblk12) -> cyemi_1399/1
  cyemi_1400/1 -> cfblk36/1
  cfblk260/1(cfblk2) -> cyemi_1400/1
  cyemi_1401/1 -> cfblk37/1
  cyemi_1402/1 -> cfblk37/2
  cyemi_1403/1 -> cfblk38/1
  cfblk290/2(cfblk13) -> cyemi_1403/1
  cyemi_1404/1 -> cfblk39/1
  cfblk30/1 -> cyemi_1404/1
  cyemi_1405/1 -> cfblk4/1
  cfblk186/1 -> cyemi_1405/1
  cyemi_1406/1 -> cfblk40/1
  cyemi_1407/1 -> cfblk41/1
  cfblk19/1 -> cyemi_1407/1
  cyemi_1408/1 -> cfblk42/1
  cfblk58/1 -> cyemi_1408/1
  cyemi_1409/1 -> cfblk43/1
  cyemi_1410/1 -> cfblk44/1
  cfblk203/1 -> cyemi_1410/1
  cyemi_1411/1 -> cfblk44/2
  cfblk78/1 -> cyemi_1411/1
  cyemi_1412/1 -> cfblk45/1
  cfblk279/1(cfblk2) -> cyemi_1412/1
  cyemi_1413/1 -> cfblk46/1
  cfblk77/1 -> cyemi_1413/1
  cyemi_1414/1 -> cfblk47/1
  cfblk82/1 -> cyemi_1414/1
  cyemi_1415/1 -> cfblk48/1
  cfblk42/1 -> cyemi_1415/1
  cyemi_1416/1 -> cfblk49/1
  cfblk22/1 -> cyemi_1416/1
  cyemi_1417/1 -> cfblk5/1
  cfblk279/2(cfblk9) -> cyemi_1417/1
  cyemi_1418/1 -> cfblk50/1
  cfblk291/2(cfblk8) -> cyemi_1418/1
  cyemi_1419/1 -> cfblk51/1
  cfblk275/1(cfblk2) -> cyemi_1419/1
  cyemi_1420/1 -> cfblk52/1
  cyemi_1421/1 -> cfblk53/1
  cfblk43/1 -> cyemi_1421/1
  cyemi_1422/1 -> cfblk54/1
  cfblk12/1 -> cyemi_1422/1
  cyemi_1423/1 -> cfblk55/1
  cfblk1/1 -> cyemi_1423/1
  cyemi_1424/1 -> cfblk56/1
  cfblk195/1 -> cyemi_1424/1
  cyemi_1425/1 -> cfblk56/2
  cfblk167/1 -> cyemi_1425/1
  cyemi_1426/1 -> cfblk57/1
  cfblk76/1 -> cyemi_1426/1
  cyemi_1427/1 -> cfblk58/1
  cfblk262/1(cfblk2) -> cyemi_1427/1
  cyemi_1428/1 -> cfblk59/1
  cfblk185/1 -> cyemi_1428/1
  cyemi_1429/1 -> cfblk6/1
  cfblk278/2(cfblk11) -> cyemi_1429/1
  cyemi_1430/1 -> cfblk60/1
  cfblk193/1 -> cyemi_1430/1
  cyemi_1431/1 -> cfblk60/2
  cyemi_1432/1 -> cfblk61/1
  cyemi_1433/1 -> cfblk62/1
  cfblk213/1 -> cyemi_1433/1
  cyemi_1434/1 -> cfblk63/1
  cfblk284/1(cfblk2) -> cyemi_1434/1
  cyemi_1435/1 -> cfblk64/1
  cyemi_1436/1 -> cfblk65/1
  cyemi_1437/1 -> cfblk66/1
  cfblk49/1 -> cyemi_1437/1
  cyemi_1438/1 -> cfblk67/1
  cfblk263/1(cfblk2) -> cyemi_1438/1
  cyemi_1439/1 -> cfblk67/2
  cfblk85/1 -> cyemi_1439/1
  cyemi_1440/1 -> cfblk68/1
  cyemi_1441/1 -> cfblk68/2
  cyemi_1442/1 -> cfblk69/1
  cyemi_1443/1 -> cfblk7/1
  cyemi_1444/1 -> cfblk70/1
  cfblk189/1 -> cyemi_1444/1
  cyemi_1445/1 -> cfblk71/1
  cfblk24/1 -> cyemi_1445/1
  cyemi_1446/1 -> cfblk71/2
  cyemi_1447/1 -> cfblk72/1
  cfblk312/1 -> cyemi_1447/1
  cyemi_1448/1 -> cfblk72/2
  cfblk289/1(cfblk2) -> cyemi_1448/1
  cyemi_1449/1 -> cfblk73/1
  cfblk68/1 -> cyemi_1449/1
  cyemi_1450/1 -> cfblk74/1
  cfblk31/1 -> cyemi_1450/1
  cyemi_1451/1 -> cfblk75/1
  cfblk246/1(cfblk2) -> cyemi_1451/1
  cyemi_1452/1 -> cfblk76/1
  cyemi_1453/1 -> cfblk76/2
  cfblk267/3(cfblk15) -> cyemi_1453/1
  cyemi_1454/1 -> cfblk77/1
  cfblk295/1(cfblk2) -> cyemi_1454/1
  cyemi_1455/1 -> cfblk78/1
  cfblk249/2(cfblk16) -> cyemi_1455/1
  cyemi_1456/1 -> cfblk79/1
  cfblk290/1(cfblk2) -> cyemi_1456/1
  cyemi_1457/1 -> cfblk8/1
  cfblk335/1 -> cyemi_1457/1
  cyemi_1458/1 -> cfblk8/2
  cfblk297/1(cfblk2) -> cyemi_1458/1
  cyemi_1459/1 -> cfblk80/1
  cyemi_1460/1 -> cfblk81/1
  cfblk245/1(cfblk2) -> cyemi_1460/1
  cyemi_1461/1 -> cfblk82/1
  cfblk18/1 -> cyemi_1461/1
  cyemi_1462/1 -> cfblk83/1
  cfblk67/1 -> cyemi_1462/1
  cyemi_1463/1 -> cfblk84/1
  cfblk270/2(cfblk10) -> cyemi_1463/1
  cyemi_1464/1 -> cfblk85/1
  cfblk41/1 -> cyemi_1464/1
  cyemi_1465/1 -> cfblk86/1
  cfblk296/2(cfblk16) -> cyemi_1465/1
  cyemi_1466/1 -> cfblk87/1
  cfblk274/1(cfblk2) -> cyemi_1466/1
  cyemi_1467/1 -> cfblk88/1
  cfblk92/1 -> cyemi_1467/1
  cyemi_1468/1 -> cfblk89/1
  cyemi_1469/1 -> cfblk9/1
  cfblk272/2(cfblk10) -> cyemi_1469/1
  cyemi_1470/1 -> cfblk90/1
  cfblk265/1(cfblk2) -> cyemi_1470/1
  cyemi_1471/1 -> cfblk91/1
  cyemi_1472/1 -> cfblk92/1
  cyemi_1473/1 -> cfblk92/2
  cfblk290/3(cfblk14) -> cyemi_1473/1
  cyemi_1474/1 -> cfblk93/1
  cfblk209/1 -> cyemi_1474/1
  cyemi_1475/1 -> cfblk94/1
  cfblk215/1 -> cyemi_1475/1
  cyemi_1476/1 -> cfblk95/1
  cyemi_1477/1 -> cfblk96/1
  cfblk65/1 -> cyemi_1477/1
  cyemi_1478/1 -> cfblk97/1
  cfblk8/1 -> cyemi_1478/1
  cyemi_1479/1 -> cfblk98/1
  cfblk17/1 -> cyemi_1479/1
  cyemi_1480/1 -> cfblk99/1
  cfblk36/1 -> cyemi_1480/1

== system sampleModel7126_pp_difftest/cfblk245 ==
  cfblk1 : Inport
  cfblk11 : Inport  Port=2
  cfblk12 : Inport  Port=3
  cfblk13 : Inport  Port=4
  cfblk14 : Inport  Port=5
  cfblk15 : Inport  Port=6
  Action Port : ActionPort  ActionType=then
  cfblk10 : If  SampleTime=1
  cfblk18 : Subsystem  TreatAsAtomicUnit=on
  cfblk19 : Subsystem  TreatAsAtomicUnit=on
  cfblk20 : Delay
  cfblk21 : DataTypeConversion  OutDataTypeStr=double
  cfblk3 : DiscreteIntegrator  SampleTime=-1  OutDataTypeStr=double  ICPrevOutput=DiscIntNeverNeededParam  ICPrevScaledInput=DiscIntNeverNeededParam
  cfblk4 : UnitDelay  SampleTime=-1
  cfblk5 : DiscreteZeroPole  Poles=[0 0.5]  Gain=1  SampleTime=-1
  cfblk6 : DiscreteFilter
  cfblk7 : simulink/Discrete/Transfer Fcn Real Zero  ZeroZ=0.75  ICPrevInput=0.0  DoSatur=off
      settings: SourceProductName=Simulink  SourceProductBaseCode=SL
  cfblk8 : simulink/Discrete/Tapped Delay  vinit=0.0  samptime=-1  NumDelays=1  DelayOrder=Oldest  includeCurrent=off
  cfblk9 : Delay
  cyemi_{68..70,79,90,92..98} (12 alike) : DataTypeConversion  OutDataTypeStr=double
  cyemi_91 : DataTypeConversion  OutDataTypeStr=fixdt('ufix32_En8')
  cfblk2 : Outport
  cfblk16 : Outport  Port=2
  cfblk17 : Outport  Port=3
  wires:
  cfblk4/1 -> cfblk16/1
  cfblk14/1 -> cfblk2/1
  cfblk18/3(cfblk11) -> cfblk17/1
  cfblk10/1 -> cfblk18/Action
  cfblk10/2 -> cfblk19/Action
  cyemi_68/1 -> cfblk10/1
  cfblk11/1 -> cyemi_68/1
  cyemi_69/1 -> cfblk18/1(cfblk1)
  cfblk15/1 -> cyemi_69/1
  cyemi_70/1 -> cfblk18/2(cfblk9)
  cfblk19/3(cfblk12) -> cyemi_70/1
  cyemi_79/1 -> cfblk19/1(cfblk1)
  cfblk3/1 -> cyemi_79/1
  cyemi_90/1 -> cfblk20/1
  cfblk18/2(cfblk10) -> cyemi_90/1
  cyemi_91/1 -> cfblk21/1
  cfblk1/1 -> cyemi_91/1
  cyemi_92/1 -> cfblk3/1
  cfblk20/1 -> cyemi_92/1
  cyemi_93/1 -> cfblk4/1
  cfblk7/1 -> cyemi_93/1
  cyemi_94/1 -> cfblk5/1
  cfblk21/1 -> cyemi_94/1
  cyemi_95/1 -> cfblk6/1
  cfblk19/1(cfblk2) -> cyemi_95/1
  cyemi_96/1 -> cfblk7/1
  cfblk18/1(cfblk2) -> cyemi_96/1
  cyemi_97/1 -> cfblk8/1
  cfblk19/2(cfblk11) -> cyemi_97/1
  cyemi_98/1 -> cfblk9/1
  cfblk8/1 -> cyemi_98/1

== system sampleModel7126_pp_difftest/cfblk246 ==
  cfblk1 : Inport
  cfblk8 : Inport  Port=2
  Action Port : ActionPort  ActionType=else
  cfblk10 : Subsystem  TreatAsAtomicUnit=on
  cfblk11 : Delay
  cfblk3 : DiscreteFilter
  cfblk4 : DiscreteStateSpace  SampleTime=-1
  cfblk5 : simulink/Discrete/Transfer Fcn Lead or Lag  PoleZ=0.95  ZeroZ=0.75  ICPrevOutput=0.0  ICPrevInput=0.0  DoSatur=off
      settings: SourceProductName=Simulink  SourceProductBaseCode=SL
  cfblk6 : simulink/Discrete/Transfer Fcn Lead or Lag  PoleZ=0.95  ZeroZ=0.75  ICPrevOutput=0.0  ICPrevInput=0.0  DoSatur=off
      settings: SourceProductName=Simulink  SourceProductBaseCode=SL
  cfblk7 : If  SampleTime=1
  cfblk9 : Subsystem  TreatAsAtomicUnit=on
  cyemi_{101..102,118..124} (9 alike) : DataTypeConversion  OutDataTypeStr=double
  cfblk2 : Outport
  wires:
  cfblk6/1 -> cfblk2/1
  cfblk7/1 -> cfblk9/Action
  cfblk7/2 -> cfblk10/Action
  cyemi_101/1 -> cfblk10/1(cfblk1)
  cfblk11/1 -> cyemi_101/1
  cyemi_102/1 -> cfblk10/2(cfblk13)
  cfblk8/1 -> cyemi_102/1
  cyemi_118/1 -> cfblk11/1
  cfblk4/1 -> cyemi_118/1
  cyemi_119/1 -> cfblk3/1
  cfblk1/1 -> cyemi_119/1
  cyemi_120/1 -> cfblk4/1
  cfblk10/1(cfblk2) -> cyemi_120/1
  cyemi_121/1 -> cfblk5/1
  cfblk3/1 -> cyemi_121/1
  cyemi_122/1 -> cfblk6/1
  cfblk10/3(cfblk15) -> cyemi_122/1
  cyemi_123/1 -> cfblk7/1
  cfblk5/1 -> cyemi_123/1
  cyemi_124/1 -> cfblk9/1(cfblk1)
  cfblk10/2(cfblk14) -> cyemi_124/1

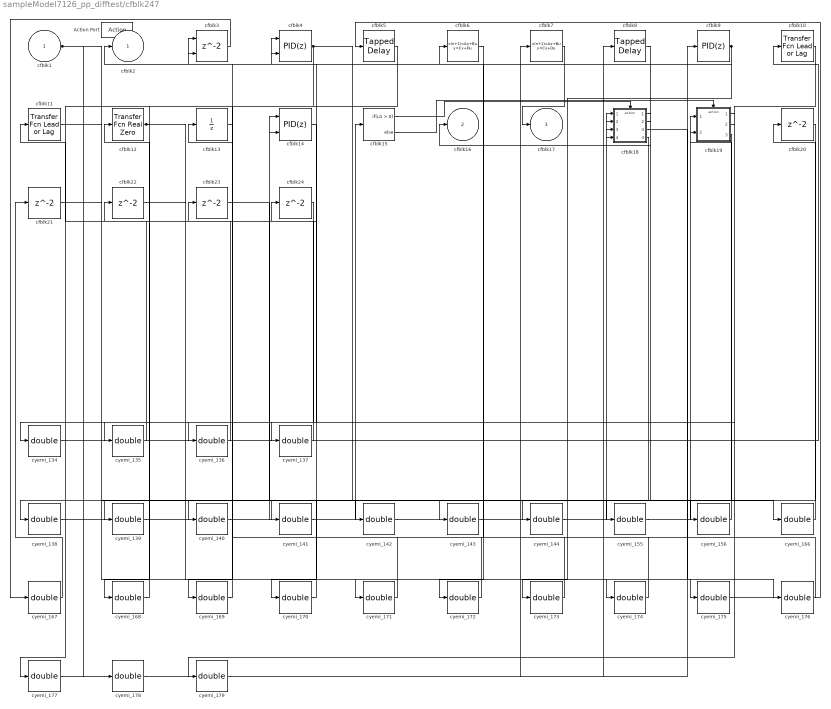
== system sampleModel7126_pp_difftest/cfblk247 ==
  cfblk1 : Inport
  Action Port : ActionPort  ActionType=then
  cfblk10 : simulink/Discrete/Transfer Fcn Lead or Lag  PoleZ=0.95  ZeroZ=0.75  ICPrevOutput=0.0  ICPrevInput=0.0  DoSatur=off
      settings: SourceProductName=Simulink  SourceProductBaseCode=SL
  cfblk11 : simulink/Discrete/Transfer Fcn Lead or Lag  PoleZ=0.95  ZeroZ=0.75  ICPrevOutput=0.0  ICPrevInput=0.0  DoSatur=off
      settings: SourceProductName=Simulink  SourceProductBaseCode=SL
  cfblk12 : simulink/Discrete/Transfer Fcn Real Zero  ZeroZ=0.75  ICPrevInput=0.0  DoSatur=off
      settings: SourceProductName=Simulink  SourceProductBaseCode=SL
  cfblk13 : UnitDelay  SampleTime=-1
  cfblk14 : simulink/Continuous/PID Controller (2DOF)  Controller=PID  TimeDomain=Discrete-time  SampleTime=-1  IntegratorMethod=Forward Euler  FilterMethod=Forward Euler  Form=Parallel  UseFilter=on  ControllerParametersSource=internal  P=1  I=1  D=0  N=100  b=1  c=1  InitialConditionSource=internal  InitialConditionForIntegrator=0  InitialConditionForFilter=0  ExternalReset=none  LimitOutput=off  UpperSaturationLimit=inf  LowerSaturationLimit=-inf  LinearizeAsGain=off  AntiWindupMode=none  Kb=1  TrackingMode=off  Kt=1  PParamMin=[]  PParamMax=[]  IParamMin=[]  IParamMax=[]  DParamMin=[]  DParamMax=[]  NParamMin=[]  NParamMax=[]  bParamMin=[]  bParamMax=[]  cParamMin=[]  cParamMax=[]  KbParamMin=[]  KbParamMax=[]  KtParamMin=[]  KtParamMax=[]  POutMin=[]  POutMax=[]  IOutMin=[]  IOutMax=[]  DOutMin=[]  DOutMax=[]  NOutMin=[]  NOutMax=[]  bOutMin=[]  bOutMax=[]  cOutMin=[]  cOutMax=[]  KbOutMin=[]  KbOutMax=[]  KtOutMin=[]  KtOutMax=[]  IntegratorOutMin=[]  IntegratorOutMax=[]  FilterOutMin=[]  FilterOutMax=[]  SumOutMin=[]  SumOutMax=[]  Sum1OutMin=[]  Sum1OutMax=[]  Sum2OutMin=[]  Sum2OutMax=[]  Sum3OutMin=[]  Sum3OutMax=[]  SumI1OutMin=[]  SumI1OutMax=[]  SumI2OutMin=[]  SumI2OutMax=[]  SumI3OutMin=[]  SumI3OutMax=[]  SumDOutMin=[]  SumDOutMax=[]  SaturationOutMin=[]  SaturationOutMax=[]  IntegratorContinuousStateAttributes=''  IntegratorStateMustResolveToSignalObject=off  IntegratorRTWStateStorageClass=Auto  FilterContinuousStateAttributes=''  FilterStateMustResolveToSignalObject=off  FilterRTWStateStorageClass=Auto  DifferentiatorICPrevScaledInput=0  DifferentiatorOutMin=[]  DifferentiatorOutMax=[]  FilterDiffOutCoefMin=[]  FilterDiffOutCoefMax=[]  SumDenOutMin=[]  SumDenOutMax=[]  SumNumOutMin=[]  SumNumOutMax=[]  ReciprocalOutMin=[]  ReciprocalOutMax=[]  DivideOutMin=[]  DivideOutMax=[]  TunerSelectOption=Transfer Function Based (PID Tuner App)
  cfblk15 : If  SampleTime=1
  cfblk18 : Subsystem  TreatAsAtomicUnit=on
  cfblk19 : Subsystem  TreatAsAtomicUnit=on
  cfblk{20..24} (5 alike) : Delay
  cfblk3 : Delay  ShowEnablePort=on
      settings: InputPortMap=u0,e6
  cfblk4 : simulink/Continuous/PID Controller (2DOF)  Controller=PID  TimeDomain=Discrete-time  SampleTime=-1  IntegratorMethod=Forward Euler  FilterMethod=Forward Euler  Form=Parallel  UseFilter=on  ControllerParametersSource=internal  P=1  I=1  D=0  N=100  b=1  c=1  InitialConditionSource=internal  InitialConditionForIntegrator=0  InitialConditionForFilter=0  ExternalReset=none  LimitOutput=off  UpperSaturationLimit=inf  LowerSaturationLimit=-inf  LinearizeAsGain=off  AntiWindupMode=none  Kb=1  TrackingMode=off  Kt=1  PParamMin=[]  PParamMax=[]  IParamMin=[]  IParamMax=[]  DParamMin=[]  DParamMax=[]  NParamMin=[]  NParamMax=[]  bParamMin=[]  bParamMax=[]  cParamMin=[]  cParamMax=[]  KbParamMin=[]  KbParamMax=[]  KtParamMin=[]  KtParamMax=[]  POutMin=[]  POutMax=[]  IOutMin=[]  IOutMax=[]  DOutMin=[]  DOutMax=[]  NOutMin=[]  NOutMax=[]  bOutMin=[]  bOutMax=[]  cOutMin=[]  cOutMax=[]  KbOutMin=[]  KbOutMax=[]  KtOutMin=[]  KtOutMax=[]  IntegratorOutMin=[]  IntegratorOutMax=[]  FilterOutMin=[]  FilterOutMax=[]  SumOutMin=[]  SumOutMax=[]  Sum1OutMin=[]  Sum1OutMax=[]  Sum2OutMin=[]  Sum2OutMax=[]  Sum3OutMin=[]  Sum3OutMax=[]  SumI1OutMin=[]  SumI1OutMax=[]  SumI2OutMin=[]  SumI2OutMax=[]  SumI3OutMin=[]  SumI3OutMax=[]  SumDOutMin=[]  SumDOutMax=[]  SaturationOutMin=[]  SaturationOutMax=[]  IntegratorContinuousStateAttributes=''  IntegratorStateMustResolveToSignalObject=off  IntegratorRTWStateStorageClass=Auto  FilterContinuousStateAttributes=''  FilterStateMustResolveToSignalObject=off  FilterRTWStateStorageClass=Auto  DifferentiatorICPrevScaledInput=0  DifferentiatorOutMin=[]  DifferentiatorOutMax=[]  FilterDiffOutCoefMin=[]  FilterDiffOutCoefMax=[]  SumDenOutMin=[]  SumDenOutMax=[]  SumNumOutMin=[]  SumNumOutMax=[]  ReciprocalOutMin=[]  ReciprocalOutMax=[]  DivideOutMin=[]  DivideOutMax=[]  TunerSelectOption=Transfer Function Based (PID Tuner App)
  cfblk5 : simulink/Discrete/Tapped Delay  vinit=0.0  samptime=-1  NumDelays=1  DelayOrder=Oldest  includeCurrent=off
  cfblk6 : DiscreteStateSpace  SampleTime=-1
  cfblk7 : DiscreteStateSpace  SampleTime=-1
  cfblk8 : simulink/Discrete/Tapped Delay  vinit=0.0  samptime=-1  NumDelays=1  DelayOrder=Oldest  includeCurrent=off
  cfblk9 : simulink/Continuous/PID Controller  Controller=PID  TimeDomain=Discrete-time  SampleTime=-1  IntegratorMethod=Forward Euler  FilterMethod=Forward Euler  Form=Parallel  UseFilter=on  ControllerParametersSource=internal  P=1  I=1  D=0  N=100  InitialConditionSource=internal  InitialConditionForIntegrator=0  InitialConditionForFilter=0  ExternalReset=none  LimitOutput=off  UpperSaturationLimit=inf  LowerSaturationLimit=-inf  LinearizeAsGain=off  AntiWindupMode=none  Kb=1  TrackingMode=off  Kt=1  PParamMin=[]  PParamMax=[]  IParamMin=[]  IParamMax=[]  DParamMin=[]  DParamMax=[]  NParamMin=[]  NParamMax=[]  KbParamMin=[]  KbParamMax=[]  KtParamMin=[]  KtParamMax=[]  POutMin=[]  POutMax=[]  IOutMin=[]  IOutMax=[]  DOutMin=[]  DOutMax=[]  NOutMin=[]  NOutMax=[]  KbOutMin=[]  KbOutMax=[]  KtOutMin=[]  KtOutMax=[]  IntegratorOutMin=[]  IntegratorOutMax=[]  FilterOutMin=[]  FilterOutMax=[]  SumOutMin=[]  SumOutMax=[]  SumI1OutMin=[]  SumI1OutMax=[]  SumI2OutMin=[]  SumI2OutMax=[]  SumI3OutMin=[]  SumI3OutMax=[]  SumDOutMin=[]  SumDOutMax=[]  SaturationOutMin=[]  SaturationOutMax=[]  IntegratorContinuousStateAttributes=''  IntegratorStateMustResolveToSignalObject=off  IntegratorRTWStateStorageClass=Auto  FilterContinuousStateAttributes=''  FilterStateMustResolveToSignalObject=off  FilterRTWStateStorageClass=Auto  DifferentiatorICPrevScaledInput=0  DifferentiatorOutMin=[]  DifferentiatorOutMax=[]  FilterDiffOutCoefMin=[]  FilterDiffOutCoefMax=[]  SumDenOutMin=[]  SumDenOutMax=[]  SumNumOutMin=[]  SumNumOutMax=[]  ReciprocalOutMin=[]  ReciprocalOutMax=[]  DivideOutMin=[]  DivideOutMax=[]  TunerSelectOption=Transfer Function Based (PID Tuner App)
  cyemi_{134..144,155..156,166..179} (27 alike) : DataTypeConversion  OutDataTypeStr=double
  cfblk2 : Outport
  cfblk16 : Outport  Port=2
  cfblk17 : Outport  Port=3
  wires:
  cfblk1/1 -> cyemi_174/1, cyemi_178/1
  cfblk12/1 -> cyemi_168/1, cyemi_171/1
  cfblk18/2(cfblk14) -> cfblk16/1
  cfblk7/1 -> cfblk17/1
  cfblk9/1 -> cfblk2/1, cyemi_173/1
  cfblk4/1 -> cyemi_139/1, cyemi_166/1, cyemi_169/1
  cfblk15/1 -> cfblk18/Action
  cfblk15/2 -> cfblk19/Action
  cyemi_134/1 -> cfblk10/1
  cfblk19/1(cfblk2) -> cyemi_134/1
  cyemi_135/1 -> cfblk11/1
  cfblk18/1(cfblk2) -> cyemi_135/1
  cyemi_136/1 -> cfblk12/1
  cfblk13/1 -> cyemi_136/1
  cyemi_137/1 -> cfblk13/1
  cfblk14/1 -> cyemi_137/1
  cyemi_138/1 -> cfblk14/1
  cfblk5/1 -> cyemi_138/1
  cyemi_139/1 -> cfblk14/2
  cyemi_140/1 -> cfblk15/1
  cfblk24/1 -> cyemi_140/1
  cyemi_141/1 -> cfblk18/1(cfblk1)
  cfblk20/1 -> cyemi_141/1
  cyemi_142/1 -> cfblk18/2(cfblk11)
  cfblk19/2(cfblk12) -> cyemi_142/1
  cyemi_143/1 -> cfblk18/3(cfblk12)
  cfblk22/1 -> cyemi_143/1
  cyemi_144/1 -> cfblk18/4(cfblk13)
  cfblk23/1 -> cyemi_144/1
  cyemi_155/1 -> cfblk19/1(cfblk1)
  cfblk8/1 -> cyemi_155/1
  cyemi_156/1 -> cfblk19/2(cfblk11)
  cfblk21/1 -> cyemi_156/1
  cyemi_166/1 -> cfblk20/1
  cyemi_167/1 -> cfblk21/1
  cfblk3/1 -> cyemi_167/1
  cyemi_168/1 -> cfblk22/1
  cyemi_169/1 -> cfblk23/1
  cyemi_170/1 -> cfblk24/1
  cfblk19/3(cfblk13) -> cyemi_170/1
  cyemi_171/1 -> cfblk3/1
  cyemi_172/1 -> cfblk3/2
  cfblk6/1 -> cyemi_172/1
  cyemi_173/1 -> cfblk4/1
  cyemi_174/1 -> cfblk4/2
  cyemi_175/1 -> cfblk5/1
  cfblk11/1 -> cyemi_175/1
  cyemi_176/1 -> cfblk6/1
  cfblk18/3(cfblk15) -> cyemi_176/1
  cyemi_177/1 -> cfblk7/1
  cfblk18/4(cfblk16) -> cyemi_177/1
  cyemi_178/1 -> cfblk8/1
  cyemi_179/1 -> cfblk9/1
  cfblk10/1 -> cyemi_179/1
